simulink model "untitled"  (R2014a)
settings: Solver=ode3  StartTime=0.0  StopTime=10.0  RelTol=1e-3
undefined symbols (not defined in the file or in its folder): Ts
libraries: arduino_io_lib x4
settings Model: Creator=omar_  LastModifiedBy=omar_
settings SolverCC: AutoInsertRateTranBlk=on

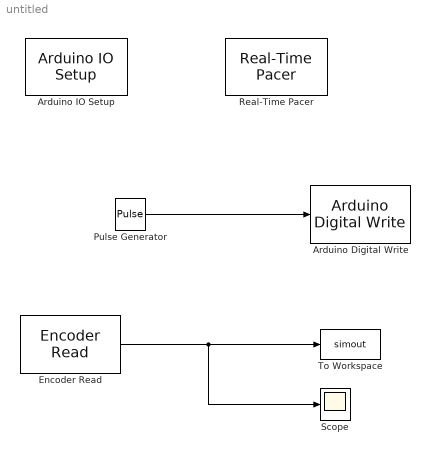
== system untitled ==
  Arduino Digital Write : arduino_io_lib/Arduino Digital Write  arduinoVar=Temporary arduino variable: Arduino1  arduinoPin=4  T=0.2
  Arduino IO Setup : arduino_io_lib/Arduino IO Setup  Priority=3  arduinoVar=Temporary arduino variable: Arduino1  workspaceVarName=a  comPort=COM12
  Encoder Read : arduino_io_lib/Encoder Read  arduinoVar=Temporary arduino variable: Arduino1  encNum=1  pinA=3  pinB=2  DbDl=0  T=Ts
  Pulse Generator : DiscretePulseGenerator  PulseType=Time based  Period=28/Ts  PulseWidth=80  PhaseDelay=2/Ts
  Real-Time Pacer : arduino_io_lib/Real-Time Pacer  simTimePerRealTime=1
  Scope : Scope
  To Workspace : ToWorkspace  VariableName=simout  SaveFormat=Timeseries  SampleTime=-1
  wires:
  Encoder Read/1 -> Scope/1, To Workspace/1
  Pulse Generator/1 -> Arduino Digital Write/1
